simulink model "HRBModel_en"  (R2021b)
settings: Solver=VariableStepAuto  StartTime=0.0  StopTime=10.0  RelTol=1e-3
values from neighbouring files (symbols this model uses):
  A = 7.20598    [HRBData.sldd]    (also in HRBModelParam.m = 7.20598)
  A_Tank = 0.25    [HRBData.sldd]    (also in HRBModelParam.m = 0.25)
  act_time = 2.0    [HRBData.sldd]    (also in HRBModelParam.m = 10)
  alpha = 0.0    [HRBData.sldd]    (also in HRBModelParam.m = deg2rad(0))
  Cd = 0.8    [HRBData.sldd]    (also in HRBModelParam.m = 0.8)
  Cr = 0.018    [HRBData.sldd]    (also in HRBModelParam.m = 0.018)
  DV = 80.0    [HRBData.sldd]    (also in HRBModelParam.m = 80)
  g = 9.81    [HRBData.sldd]    (also in HRBModelParam.m = 9.81)
  gamma = 1.4    [HRBData.sldd]    (also in HRBModelParam.m = 1.4)
  ilk_hiz = 15.0    [HRBData.sldd]    (also in HRBModelParam.m = 0)
  m = 18000.0    [HRBData.sldd]    (also in HRBModelParam.m = 18000)
  mech_eff = 0.9    [HRBData.sldd]    (also in HRBModelParam.m = 0.9)
  mu_AT = 0.8    [HRBData.sldd]    (also in HRBModelParam.m = 0.8)
  mu_HA = 0.8    [HRBData.sldd]    (also in HRBModelParam.m = 0.8)
  P0 = 50.0    [HRBData.sldd]    (also in HRBModelParam.m = 50)
  P1 = 60.0    [HRBData.sldd]    (also in HRBModelParam.m = 395)
  Patm = 1.0    [HRBData.sldd]    (also in HRBModelParam.m = 1)
  Pmax = 400.0    [HRBData.sldd]    (also in HRBModelParam.m = 400)
  r = 0.5715    [HRBData.sldd]    (also in HRBModelParam.m = 0.5715)
  R_AT = 4.11    [HRBData.sldd]    (also in HRBModelParam.m = 4.11)
  R_HA = 7.0    [HRBData.sldd]    (also in HRBModelParam.m = 7)
  R_PM_Aku = 0.07    [HRBData.sldd]    (also in HRBModelParam.m = 0.07)
  rho = 1.225    [HRBData.sldd]    (also in HRBModelParam.m = 1.225)
  rho_oil = 700.0    [HRBData.sldd]    (also in HRBModelParam.m = 700)
  V0 = 0.06    [HRBData.sldd]    (also in HRBModelParam.m = 0.06)
  V_oil = 0.1    [HRBData.sldd]    (also in HRBModelParam.m = 0.1)
  vol_eff = 0.9    [HRBData.sldd]    (also in HRBModelParam.m = 0.9)
libraries: simulink_extras x1
settings Model: DataDictionary=HRBData.sldd  Creator=erkin  LastModifiedBy=erkin
settings DebuggingCC: UnderspecifiedInitializationDetection=Classic  MergeDetectMultiDrivingBlocksExec=none
settings ModelReferenceCC: PropagateSignalLabelsOutOfModel=off

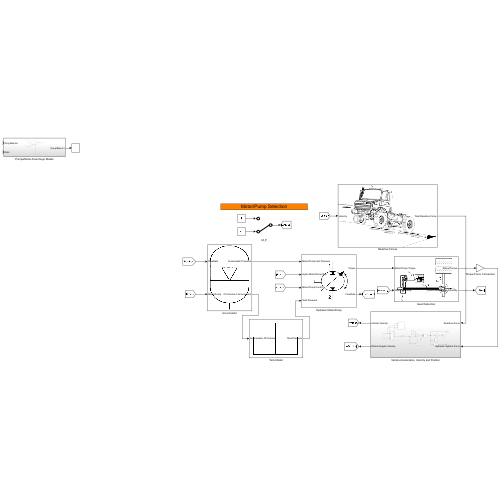
[thumbnail: Simulink's stored preview of the top-level diagram]
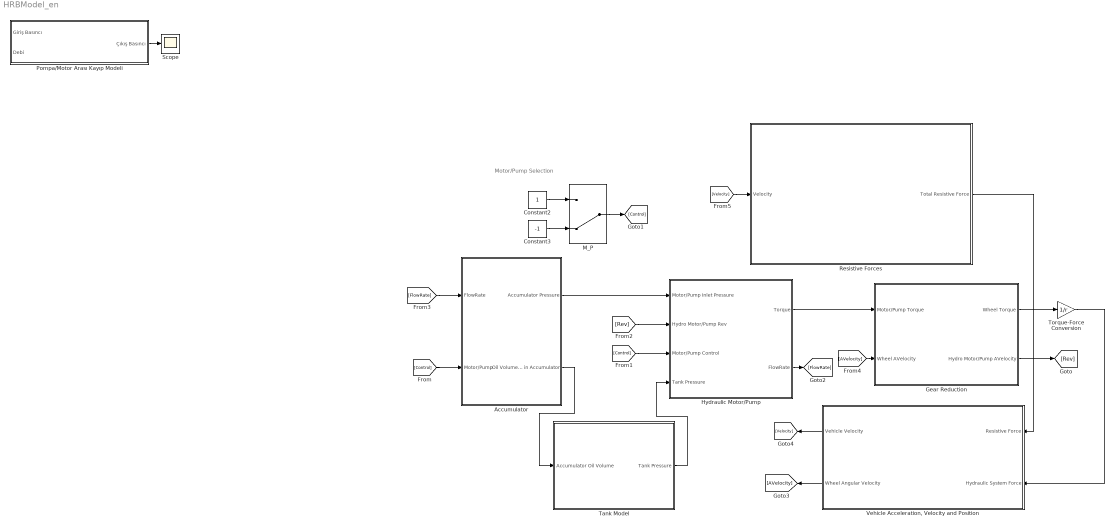
== system HRBModel_en ==
  note: Motor/Pump Selection
  Accumulator : Subsystem
      mask Display: image('$imagefile'); % Use "Edit Image" on toolstrip to change.
  Constant2 : Constant
  Constant3 : Constant  Value=-1
  Gear Reduction : Subsystem
      mask Display: image('$imagefile'); % Use "Edit Image" on toolstrip to change.
  Hydraulic Motor/Pump : Subsystem
      mask Display: image('$imagefile'); % Use "Edit Image" on toolstrip to change.
  M_P : ManualSwitch  CurrentSetting=0
  Pompa/Motor Arası Kayıp Modeli : Subsystem
  Resistive Forces : Subsystem
      mask Display: image('$imagefile'); % Use "Edit Image" on toolstrip to change.
  Scope : Scope
  Tank Model : Subsystem
      mask Display: image('$imagefile'); % Use "Edit Image" on toolstrip to change.
  Torque-Force Conversion : Gain  Gain=1/r
  "Vehicle Acceleration, Velocity and Position" : Subsystem
  wires:
  Hydraulic Motor/Pump/1(Torque) -> Gear Reduction/1(Motor/Pump Torque)
  Gear Reduction/1(Wheel Torque) -> Torque-Force Conversion/1
  Torque-Force Conversion/1 -> "Vehicle Acceleration, Velocity and Position"/2(Hydraulic System Force)
  Resistive Forces/1(Total Resistive Force) -> "Vehicle Acceleration, Velocity and Position"/1(Resistive Force)
  [Control] -> Accumulator/2(Motor/Pump)
  Constant2/1 -> M_P/1
  Constant3/1 -> M_P/2
  M_P/1 -> [Control]
  [Control] -> Hydraulic Motor/Pump/3(Motor/Pump Control)
  Tank Model/1(Tank Pressure) -> Hydraulic Motor/Pump/4(Tank Pressure)
  Accumulator/2(Oil Volume in Accumulator) -> Tank Model/1(Accumulator Oil Volume)
  Accumulator/1(Accumulator Pressure) -> Hydraulic Motor/Pump/1(Motor/Pump Inlet Pressure)
  Pompa/Motor Arası Kayıp Modeli/1(Çıkış Basıncı) -> Scope/1
  [Rev] -> Hydraulic Motor/Pump/2(Hydro Motor/Pump Rev)
  Gear Reduction/2(Hydro Motor/Pump AVelocity) -> [Rev]
  [FlowRate] -> Accumulator/1(FlowRate)
  Hydraulic Motor/Pump/2(FlowRate) -> [FlowRate]
  "Vehicle Acceleration, Velocity and Position"/2(Wheel Angular Velocity) -> [AVelocity]
  [AVelocity] -> Gear Reduction/2(Wheel AVelocity)
  [Velocity] -> Resistive Forces/1(Velocity)
  "Vehicle Acceleration, Velocity and Position"/1(Vehicle Velocity) -> [Velocity]

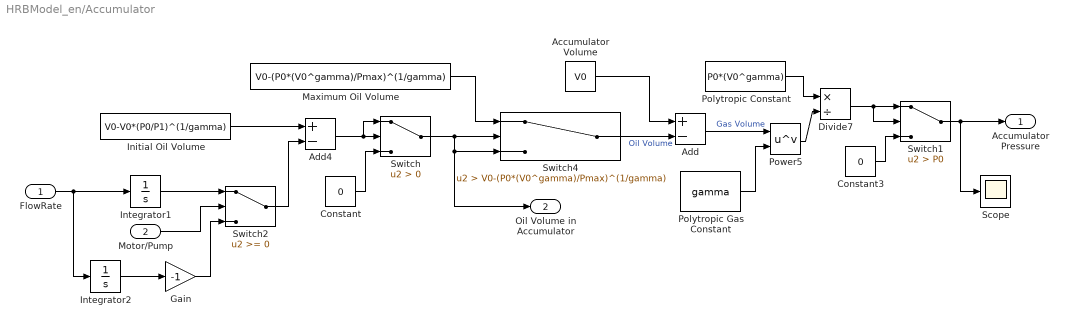
== system HRBModel_en/Accumulator ==
  FlowRate : Inport
  Motor/Pump : Inport  Port=2
  Accumulator Volume : Constant  Value=V0
  Add : Sum  Inputs=+-
  Add4 : Sum  Inputs=+-
  Constant : Constant  Value=0
  Constant3 : Constant  Value=0
  Divide7 : Product  Inputs=*/
  Gain : Gain  Gain=-1
  Initial Oil Volume : Constant  Value=V0-V0*(P0/P1)^(1/gamma)
  Integrator1 : Integrator
  Integrator2 : Integrator
  Maximum Oil Volume : Constant  Value=V0-(P0*(V0^gamma)/Pmax)^(1/gamma)
  Polytropic Constant : Constant  Value=P0*(V0^gamma)
  Polytropic Gas Constant : Constant  Value=gamma
  Power5 : Math  Operator=pow  SaturateOnIntegerOverflow=on
  Scope : Scope
  Switch : Switch  Criteria=u2 > Threshold
  Switch1 : Switch  Criteria=u2 > Threshold  Threshold=P0
  Switch2 : Switch
  Switch4 : Switch  Criteria=u2 > Threshold  Threshold=V0-(P0*(V0^gamma)/Pmax)^(1/gamma)
  Accumulator Pressure : Outport
  Oil Volume in Accumulator : Outport  Port=2
  wires:
  Divide7/1 -> Switch1/2, Switch1/1
  Initial Oil Volume/1 -> Add4/1
  Polytropic Constant/1 -> Divide7/1
  Switch/1 -> Oil Volume in Accumulator/1, Switch4/3, Switch4/2
  FlowRate/1 -> Integrator2/1, Integrator1/1
  Accumulator Volume/1 -> Add/1
  Add/1 -> Power5/1  "Gas Volume"
  Polytropic Gas Constant/1 -> Power5/2
  Power5/1 -> Divide7/2
  Add4/1 -> Switch/1, Switch/2
  Constant/1 -> Switch/3
  Constant3/1 -> Switch1/3
  Integrator1/1 -> Switch2/1
  Switch2/1 -> Add4/2
  Integrator2/1 -> Gain/1
  Gain/1 -> Switch2/3
  Switch1/1 -> Accumulator Pressure/1, Scope/1
  Motor/Pump/1 -> Switch2/2
  Maximum Oil Volume/1 -> Switch4/1
  Switch4/1 -> Add/2  "Oil Volume"

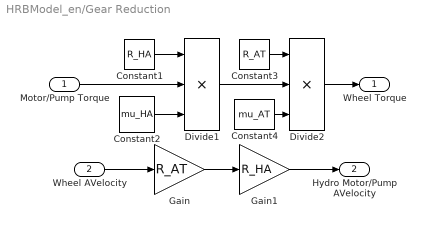
== system HRBModel_en/Gear Reduction ==
  Motor/Pump Torque : Inport
  Wheel AVelocity : Inport  Port=2
  Constant1 : Constant  Value=R_HA
  Constant2 : Constant  Value=mu_HA
  Constant3 : Constant  Value=R_AT
  Constant4 : Constant  Value=mu_AT
  Divide1 : Product  Inputs=***
  Divide2 : Product  Inputs=***
  Gain : Gain  Gain=R_AT
  Gain1 : Gain  Gain=R_HA
  Wheel Torque : Outport
  Hydro Motor/Pump AVelocity : Outport  Port=2
  wires:
  Constant3/1 -> Divide2/1
  Constant2/1 -> Divide1/3
  Divide2/1 -> Wheel Torque/1
  Constant4/1 -> Divide2/3
  Constant1/1 -> Divide1/1
  Divide1/1 -> Divide2/2
  Motor/Pump Torque/1 -> Divide1/2
  Wheel AVelocity/1 -> Gain/1
  Gain/1 -> Gain1/1
  Gain1/1 -> Hydro Motor/Pump AVelocity/1

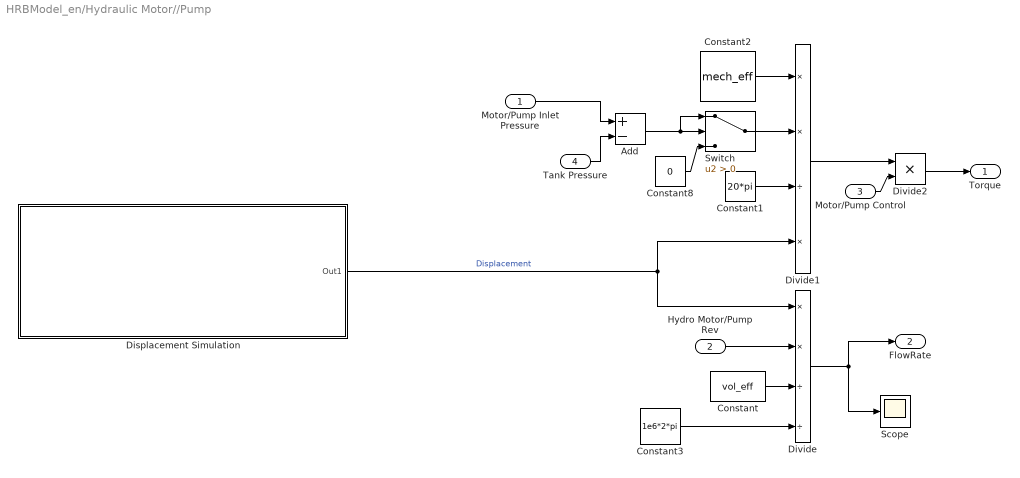
== system HRBModel_en/Hydraulic Motor//Pump ==
  Motor/Pump Inlet Pressure : Inport
  Hydro Motor/Pump Rev : Inport  Port=2
  Motor/Pump Control : Inport  Port=3
  Tank Pressure : Inport  Port=4
  Add : Sum  Inputs=+-
  Constant : Constant  Value=vol_eff
  Constant1 : Constant  Value=20*pi
  Constant2 : Constant  Value=mech_eff
  Constant3 : Constant  Value=1e6*2*pi
  Constant8 : Constant  Value=0
  Displacement Simulation : Subsystem
  Divide : Product  Inputs=**//
  Divide1 : Product  Inputs=**/*
  Divide2 : Product  Inputs=**
  Scope : Scope
  Switch : Switch  Criteria=u2 > Threshold
  Torque : Outport
  FlowRate : Outport  Port=2
  wires:
  Constant1/1 -> Divide1/3
  Motor/Pump Inlet Pressure/1 -> Add/1
  Divide1/1 -> Divide2/1
  Hydro Motor/Pump Rev/1 -> Divide/2
  Constant/1 -> Divide/3
  Divide/1 -> FlowRate/1, Scope/1
  Constant3/1 -> Divide/4
  Divide2/1 -> Torque/1
  Motor/Pump Control/1 -> Divide2/2
  Add/1 -> Switch/1, Switch/2
  Switch/1 -> Divide1/2
  Constant8/1 -> Switch/3
  Tank Pressure/1 -> Add/2
  Displacement Simulation/1(Out1) -> Divide1/4, Divide/1  "Displacement"
  Constant2/1 -> Divide1/1

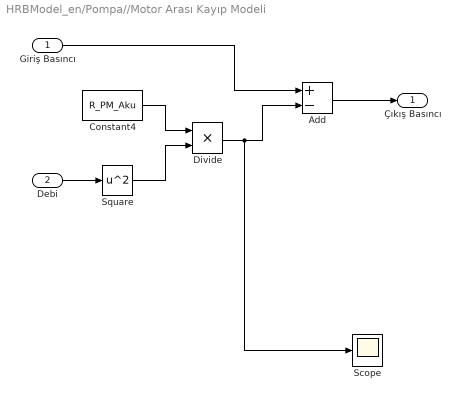
== system HRBModel_en/Pompa//Motor Arası Kayıp Modeli ==
  Giriş Basıncı : Inport
  Debi : Inport  Port=2
  Add : Sum  Inputs=+-
  Constant4 : Constant  Value=R_PM_Aku
  Divide : Product  Inputs=**
  Scope : Scope
  Square : Math  Operator=square  SaturateOnIntegerOverflow=on
  Çıkış Basıncı : Outport
  wires:
  Debi/1 -> Square/1
  Square/1 -> Divide/2
  Constant4/1 -> Divide/1
  Giriş Basıncı/1 -> Add/1
  Divide/1 -> Scope/1, Add/2
  Add/1 -> Çıkış Basıncı/1

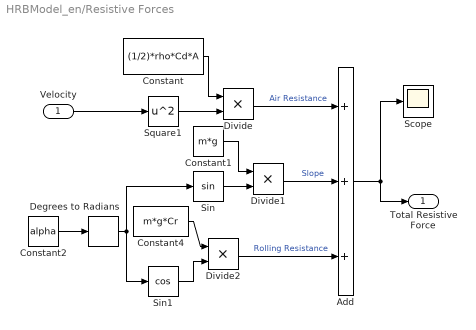
== system HRBModel_en/Resistive Forces ==
  Velocity : Inport
  Add : Sum  Inputs=+++
  Constant : Constant  Value=(1/2)*rho*Cd*A
  Constant1 : Constant  Value=m*g
  Constant2 : Constant  Value=alpha
  Constant4 : Constant  Value=m*g*Cr
  Degrees to Radians : simulink_extras/Transformations/Degrees to Radians
  Divide : Product  Inputs=**
  Divide1 : Product  Inputs=**
  Divide2 : Product  Inputs=**
  Scope : Scope
  Sin : Trigonometry
  Sin1 : Trigonometry  Operator=cos
  Square1 : Math  Operator=square  SaturateOnIntegerOverflow=on
  Total Resistive Force : Outport
  wires:
  Sin1/1 -> Divide2/2
  Divide1/1 -> Add/2  "Slope"
  Divide2/1 -> Add/3  "Rolling Resistance"
  Add/1 -> Total Resistive Force/1, Scope/1
  Velocity/1 -> Square1/1
  Constant2/1 -> Degrees to Radians/1
  Degrees to Radians/1 -> Sin1/1, Sin/1
  Square1/1 -> Divide/2
  Constant/1 -> Divide/1
  Divide/1 -> Add/1  "Air Resistance"
  Constant1/1 -> Divide1/1
  Sin/1 -> Divide1/2
  Constant4/1 -> Divide2/1

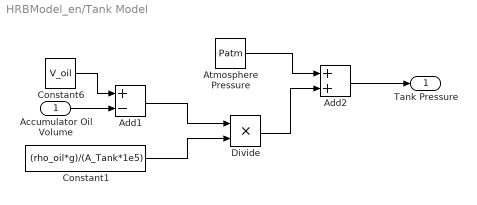
== system HRBModel_en/Tank Model ==
  Accumulator Oil Volume : Inport
  Add1 : Sum  Inputs=+-
  Add2 : Sum
  Atmosphere Pressure : Constant  Value=Patm
  Constant1 : Constant  Value=(rho_oil*g)/(A_Tank*1e5)
  Constant6 : Constant  Value=V_oil
  Divide : Product  Inputs=**
  Tank Pressure : Outport
  wires:
  Constant6/1 -> Add1/1
  Add1/1 -> Divide/1
  Accumulator Oil Volume/1 -> Add1/2
  Atmosphere Pressure/1 -> Add2/1
  Add2/1 -> Tank Pressure/1
  Constant1/1 -> Divide/2
  Divide/1 -> Add2/2

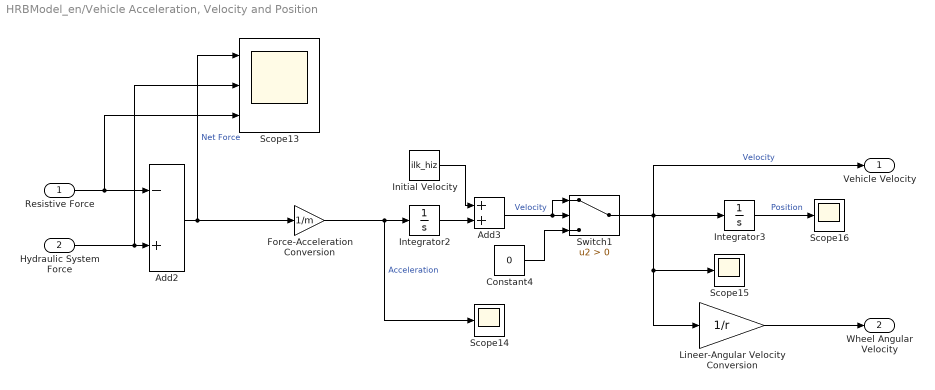
== system HRBModel_en/Vehicle Acceleration, Velocity and Position ==
  Resistive Force : Inport
  Hydraulic System Force : Inport  Port=2
  Add2 : Sum  Inputs=-+
  Add3 : Sum
  Constant4 : Constant  Value=0
  Force-Acceleration Conversion : Gain  Gain=1/m
  Initial Velocity : Constant  Value=ilk_hiz
  Integrator2 : Integrator
  Integrator3 : Integrator
  Lineer-Angular Velocity Conversion : Gain  Gain=1/r
  Scope13 : Scope  NumInputPorts=3
  Scope14 : Scope
  Scope15 : Scope
  Scope16 : Scope
  Switch1 : Switch  Criteria=u2 > Threshold
  Vehicle Velocity : Outport
  Wheel Angular Velocity : Outport  Port=2
  wires:
  Force-Acceleration Conversion/1 -> Integrator2/1, Scope14/1  "Acceleration"
  Constant4/1 -> Switch1/3
  Add2/1 -> Force-Acceleration Conversion/1, Scope13/1  "Net Force"
  Integrator2/1 -> Add3/2
  Initial Velocity/1 -> Add3/1
  Switch1/1 -> Vehicle Velocity/1, Integrator3/1, Lineer-Angular Velocity Conversion/1, Scope15/1  "Velocity"
  Integrator3/1 -> Scope16/1  "Position"
  Add3/1 -> Switch1/1, Switch1/2  "Velocity"
  Resistive Force/1 -> Scope13/3, Add2/1
  Hydraulic System Force/1 -> Scope13/2, Add2/2
  Lineer-Angular Velocity Conversion/1 -> Wheel Angular Velocity/1

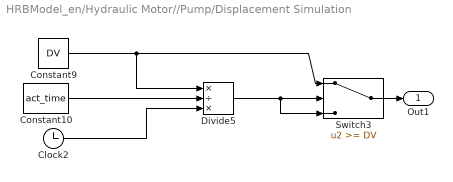
== system HRBModel_en/Hydraulic Motor//Pump/Displacement Simulation ==
  Clock2 : Clock
  Constant10 : Constant  Value=act_time
  Constant9 : Constant  Value=DV
  Divide5 : Product  Inputs=*/*
  Switch3 : Switch  Threshold=DV
  Out1 : Outport
  wires:
  Clock2/1 -> Divide5/3
  Divide5/1 -> Switch3/3, Switch3/2
  Switch3/1 -> Out1/1
  Constant9/1 -> Divide5/1, Switch3/1
  Constant10/1 -> Divide5/2
